simulink model "ACC_speed_change_curve_cs"  (R2016a)
settings: Solver=ode5  SolverMode=SingleTasking  StartTime=0.0  StopTime=inf  FixedStep=1/1000  RelTol=1e-3
PreLoadFcn:
  | mbxruntime.callbacks.PreLoadFcn(bdroot);
  | check_NUTS_defined;
  | 
  | assignin('base',['model_closed_' bdroot],false);addpath('../includes_ACC');
PostLoadFcn:
  | mbxruntime.callbacks.PostLoadFcn(bdroot);
InitFcn:
  | mbxruntime.callbacks.InitFcn(bdroot);
StartFcn:
  | mbxruntime.callbacks.StartFcn(bdroot);
StopFcn:
  | mbxruntime.callbacks.StopFcn(bdroot);
model workspace (MAT data in the model file):
  mbox_table : struct (value not decoded)
  model_closed = 0
  sim_status = 0
undefined symbols (not defined in the file or in its folder): DiscIntNeverNeededParam
undefined symbols (not defined in the file): SteeringColumn, SteeringWheel, WheelL0, WheelL1, WheelR0, WheelR1
libraries: simulink_extras x49, simulink x29, PreScanSimulinkLibrary x24, PreScanUsefulBlocks x2, Solver_SF x1, simulink_need_slupdate x1
(part 6 of 17)

== system ACC_speed_change_curve_cs/WheelR0_Audi_A8_1 ==
  WheelR0_Audi_A8_1 : Inport  Tag=inport/JointActuator  OutDataTypeStr=Bus: PRESCAN_POSE_DATA  SampleTime=20/1000  BusOutputAsStruct=on
  Actuator : Subsystem  Tag=VisuJoint  mask(PreScan Sink Block: VisuJoint){UniqueID=13, Translate_ObjectID3D=Audi_A8_1.WheelR0, Rotate_ObjectID3D=Audi_A8_1.WheelR0, TimeStep=20/1000, DisplayName=[]}
      mask prompts: UniqueID "Parent Unique ID"; Translate_ObjectID3D "Translate Object Name"; Rotate_ObjectID3D "Rotate Object Name"; TimeStep "Simulation Step"; DisplayName "Display Name"
      mask help:
      | The VisuJoint block provides a way to adapt the location and orientation of a part of an object.
      |
      | For more information, please click Help.
      settings: DeleteFcn=PreScanBlockDeleteFcn;
      mask Help: eval('openHelp(223)')
      mask Display: image(imread('Joint.png'))
  wires:
  WheelR0_Audi_A8_1/1 -> Actuator/1(Joint)

== system ACC_speed_change_curve_cs/WheelR0_BMW_X5_1 ==
  WheelR0_BMW_X5_1 : Inport  Tag=inport/JointActuator  OutDataTypeStr=Bus: PRESCAN_POSE_DATA  SampleTime=20/1000  BusOutputAsStruct=on
  Actuator : Subsystem  Tag=VisuJoint  mask(PreScan Sink Block: VisuJoint){UniqueID=18, Translate_ObjectID3D=BMW_X5_1.WheelR0, Rotate_ObjectID3D=BMW_X5_1.WheelR0, TimeStep=20/1000, DisplayName=[]}
      mask prompts: UniqueID "Parent Unique ID"; Translate_ObjectID3D "Translate Object Name"; Rotate_ObjectID3D "Rotate Object Name"; TimeStep "Simulation Step"; DisplayName "Display Name"
      mask help:
      | The VisuJoint block provides a way to adapt the location and orientation of a part of an object.
      |
      | For more information, please click Help.
      settings: DeleteFcn=PreScanBlockDeleteFcn;
      mask Help: eval('openHelp(223)')
      mask Display: image(imread('Joint.png'))
  wires:
  WheelR0_BMW_X5_1/1 -> Actuator/1(Joint)

== system ACC_speed_change_curve_cs/WheelR0_Toyota_Previa_1 ==
  WheelR0_Toyota_Previa_1 : Inport  Tag=inport/JointActuator  OutDataTypeStr=Bus: PRESCAN_POSE_DATA  SampleTime=20/1000  BusOutputAsStruct=on
  Actuator : Subsystem  Tag=VisuJoint  mask(PreScan Sink Block: VisuJoint){UniqueID=724, Translate_ObjectID3D=Toyota_Previa_1.WheelR0, Rotate_ObjectID3D=Toyota_Previa_1.WheelR0, TimeStep=20/1000, DisplayName=[]}
      mask prompts: UniqueID "Parent Unique ID"; Translate_ObjectID3D "Translate Object Name"; Rotate_ObjectID3D "Rotate Object Name"; TimeStep "Simulation Step"; DisplayName "Display Name"
      mask help:
      | The VisuJoint block provides a way to adapt the location and orientation of a part of an object.
      |
      | For more information, please click Help.
      settings: DeleteFcn=PreScanBlockDeleteFcn;
      mask Help: eval('openHelp(223)')
      mask Display: image(imread('Joint.png'))
  wires:
  WheelR0_Toyota_Previa_1/1 -> Actuator/1(Joint)

== system ACC_speed_change_curve_cs/WheelR0_Toyota_Yaris_1 ==
  WheelR0_Toyota_Yaris_1 : Inport  Tag=inport/JointActuator  OutDataTypeStr=Bus: PRESCAN_POSE_DATA  SampleTime=20/1000  BusOutputAsStruct=on
  Actuator : Subsystem  Tag=VisuJoint  mask(PreScan Sink Block: VisuJoint){UniqueID=721, Translate_ObjectID3D=Toyota_Yaris_1.WheelR0, Rotate_ObjectID3D=Toyota_Yaris_1.WheelR0, TimeStep=20/1000, DisplayName=[]}
      mask prompts: UniqueID "Parent Unique ID"; Translate_ObjectID3D "Translate Object Name"; Rotate_ObjectID3D "Rotate Object Name"; TimeStep "Simulation Step"; DisplayName "Display Name"
      mask help:
      | The VisuJoint block provides a way to adapt the location and orientation of a part of an object.
      |
      | For more information, please click Help.
      settings: DeleteFcn=PreScanBlockDeleteFcn;
      mask Help: eval('openHelp(223)')
      mask Display: image(imread('Joint.png'))
  wires:
  WheelR0_Toyota_Yaris_1/1 -> Actuator/1(Joint)

== system ACC_speed_change_curve_cs/WheelR1_Audi_A8_1 ==
  WheelR1_Audi_A8_1 : Inport  Tag=inport/JointActuator  OutDataTypeStr=Bus: PRESCAN_POSE_DATA  SampleTime=20/1000  BusOutputAsStruct=on
  Actuator : Subsystem  Tag=VisuJoint  mask(PreScan Sink Block: VisuJoint){UniqueID=13, Translate_ObjectID3D=Audi_A8_1.WheelR1, Rotate_ObjectID3D=Audi_A8_1.WheelR1, TimeStep=20/1000, DisplayName=[]}
      mask prompts: UniqueID "Parent Unique ID"; Translate_ObjectID3D "Translate Object Name"; Rotate_ObjectID3D "Rotate Object Name"; TimeStep "Simulation Step"; DisplayName "Display Name"
      mask help:
      | The VisuJoint block provides a way to adapt the location and orientation of a part of an object.
      |
      | For more information, please click Help.
      settings: DeleteFcn=PreScanBlockDeleteFcn;
      mask Help: eval('openHelp(223)')
      mask Display: image(imread('Joint.png'))
  wires:
  WheelR1_Audi_A8_1/1 -> Actuator/1(Joint)

== system ACC_speed_change_curve_cs/WheelR1_BMW_X5_1 ==
  WheelR1_BMW_X5_1 : Inport  Tag=inport/JointActuator  OutDataTypeStr=Bus: PRESCAN_POSE_DATA  SampleTime=20/1000  BusOutputAsStruct=on
  Actuator : Subsystem  Tag=VisuJoint  mask(PreScan Sink Block: VisuJoint){UniqueID=18, Translate_ObjectID3D=BMW_X5_1.WheelR1, Rotate_ObjectID3D=BMW_X5_1.WheelR1, TimeStep=20/1000, DisplayName=[]}
      mask prompts: UniqueID "Parent Unique ID"; Translate_ObjectID3D "Translate Object Name"; Rotate_ObjectID3D "Rotate Object Name"; TimeStep "Simulation Step"; DisplayName "Display Name"
      mask help:
      | The VisuJoint block provides a way to adapt the location and orientation of a part of an object.
      |
      | For more information, please click Help.
      settings: DeleteFcn=PreScanBlockDeleteFcn;
      mask Help: eval('openHelp(223)')
      mask Display: image(imread('Joint.png'))
  wires:
  WheelR1_BMW_X5_1/1 -> Actuator/1(Joint)

== system ACC_speed_change_curve_cs/WheelR1_Toyota_Previa_1 ==
  WheelR1_Toyota_Previa_1 : Inport  Tag=inport/JointActuator  OutDataTypeStr=Bus: PRESCAN_POSE_DATA  SampleTime=20/1000  BusOutputAsStruct=on
  Actuator : Subsystem  Tag=VisuJoint  mask(PreScan Sink Block: VisuJoint){UniqueID=724, Translate_ObjectID3D=Toyota_Previa_1.WheelR1, Rotate_ObjectID3D=Toyota_Previa_1.WheelR1, TimeStep=20/1000, DisplayName=[]}
      mask prompts: UniqueID "Parent Unique ID"; Translate_ObjectID3D "Translate Object Name"; Rotate_ObjectID3D "Rotate Object Name"; TimeStep "Simulation Step"; DisplayName "Display Name"
      mask help:
      | The VisuJoint block provides a way to adapt the location and orientation of a part of an object.
      |
      | For more information, please click Help.
      settings: DeleteFcn=PreScanBlockDeleteFcn;
      mask Help: eval('openHelp(223)')
      mask Display: image(imread('Joint.png'))
  wires:
  WheelR1_Toyota_Previa_1/1 -> Actuator/1(Joint)

== system ACC_speed_change_curve_cs/WheelR1_Toyota_Yaris_1 ==
  WheelR1_Toyota_Yaris_1 : Inport  Tag=inport/JointActuator  OutDataTypeStr=Bus: PRESCAN_POSE_DATA  SampleTime=20/1000  BusOutputAsStruct=on
  Actuator : Subsystem  Tag=VisuJoint  mask(PreScan Sink Block: VisuJoint){UniqueID=721, Translate_ObjectID3D=Toyota_Yaris_1.WheelR1, Rotate_ObjectID3D=Toyota_Yaris_1.WheelR1, TimeStep=20/1000, DisplayName=[]}
      mask prompts: UniqueID "Parent Unique ID"; Translate_ObjectID3D "Translate Object Name"; Rotate_ObjectID3D "Rotate Object Name"; TimeStep "Simulation Step"; DisplayName "Display Name"
      mask help:
      | The VisuJoint block provides a way to adapt the location and orientation of a part of an object.
      |
      | For more information, please click Help.
      settings: DeleteFcn=PreScanBlockDeleteFcn;
      mask Help: eval('openHelp(223)')
      mask Display: image(imread('Joint.png'))
  wires:
  WheelR1_Toyota_Yaris_1/1 -> Actuator/1(Joint)

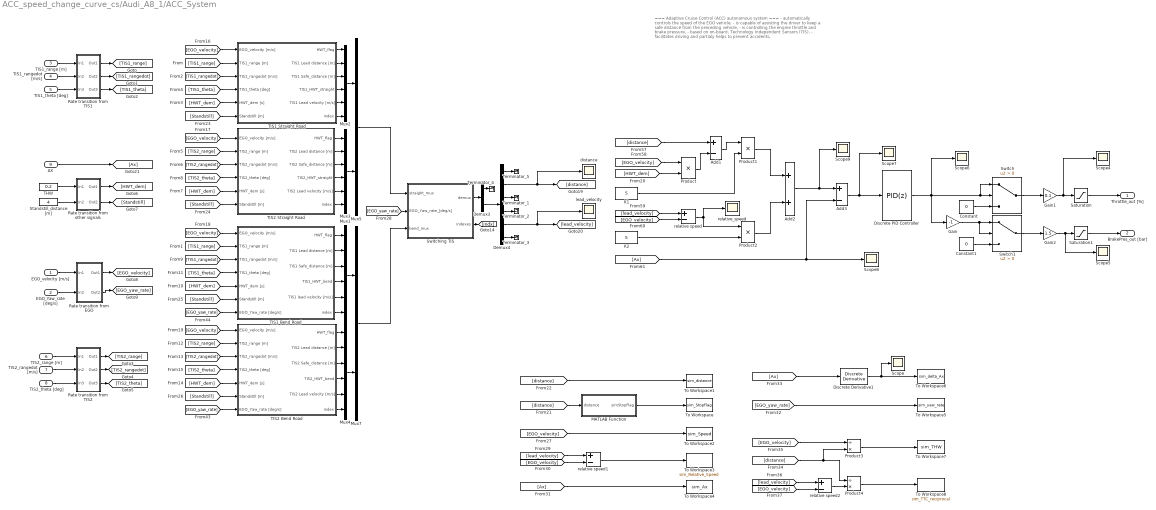
== system ACC_speed_change_curve_cs/Audi_A8_1/ACC_System ==
  note: === Adaptive Cruise Control (ACC) autonomous system ===
      |
      |  - automatically controls the speed of the EGO vehicle,
      |  - is capable of assisting the driver to keep a safe distance
      |    from the preceding vehicle,
      |  - is controlling the engine throttle and brake pressure,
      |  - based on on-board, Technology Independent Sensors (TIS),
      |  - facilitates driving and partialy helps to prevent accidents.
  EGO_velocity [m/s] : Inport  SampleTime=Tblock
  EGO_Yaw_rate [deg/s] : Inport  Port=2  SampleTime=Tblock
  TIS1_range [m] : Inport  Port=3  PortDimensions=TISdet(1)  SampleTime=TISsensor(1)
  TIS1_rangedot [m/s] : Inport  Port=4  PortDimensions=TISdet(1)  SampleTime=TISsensor(1)
  TIS1_theta [deg] : Inport  Port=5  PortDimensions=TISdet(1)  SampleTime=TISsensor(1)
  TIS2_range [m] : Inport  Port=6  PortDimensions=TISdet(2)  SampleTime=TISsensor(2)
  TIS2_rangedot [m/s] : Inport  Port=7  PortDimensions=TISdet(2)  SampleTime=TISsensor(2)
  TIS2_theta [deg] : Inport  Port=8  PortDimensions=TISdet(2)  SampleTime=TISsensor(2)
  AX : Inport  Port=9
  Add1 : Sum  Inputs=+-
  Add2 : Sum
  Add3 : Sum  Inputs=+-
  Constant : Constant  Value=0
  Constant1 : Constant  Value=0
  Demux3 : Demux  Outputs=2
  Demux4 : Demux  Outputs=6
  Discrete Derivative1 : simulink/Discrete/Discrete Derivative  gainval=1.0  ICPrevScaledInput=0.0  OutMin=[]  OutMax=[]  OutDataType=fixdt(1, 16)  OutScaling=2^-10  DoSatur=off
  Discrete PID Controller : simulink/Continuous/PID Controller  Controller=PID  TimeDomain=Discrete-time  SampleTime=-1  IntegratorMethod=Forward Euler  FilterMethod=Forward Euler  Form=Parallel  UseFilter=on  ControllerParametersSource=internal  P=50  I=5  D=0  N=100  InitialConditionSource=internal  InitialConditionForIntegrator=0  InitialConditionForFilter=0  ExternalReset=none  LimitOutput=off  UpperSaturationLimit=inf  LowerSaturationLimit=-inf  LinearizeAsGain=off  AntiWindupMode=none  Kb=1  TrackingMode=off  Kt=1  PParamMin=[]  PParamMax=[]  IParamMin=[]  IParamMax=[]  DParamMin=[]  DParamMax=[]  NParamMin=[]  NParamMax=[]  KbParamMin=[]  KbParamMax=[]  KtParamMin=[]  KtParamMax=[]  POutMin=[]  POutMax=[]  IOutMin=[]  IOutMax=[]  DOutMin=[]  DOutMax=[]  NOutMin=[]  NOutMax=[]  KbOutMin=[]  KbOutMax=[]  KtOutMin=[]  KtOutMax=[]  IntegratorOutMin=[]  IntegratorOutMax=[]  FilterOutMin=[]  FilterOutMax=[]  SumOutMin=[]  SumOutMax=[]  SumI1OutMin=[]  SumI1OutMax=[]  SumI2OutMin=[]  SumI2OutMax=[]  SumI3OutMin=[]  SumI3OutMax=[]  SumDOutMin=[]  SumDOutMax=[]  SaturationOutMin=[]  SaturationOutMax=[]  IntegratorContinuousStateAttributes=''  IntegratorStateMustResolveToSignalObject=off  IntegratorRTWStateStorageClass=Auto  FilterContinuousStateAttributes=''  FilterStateMustResolveToSignalObject=off  FilterRTWStateStorageClass=Auto  DifferentiatorICPrevScaledInput=0  DifferentiatorOutMin=[]  DifferentiatorOutMax=[]
  Gain : Gain  Gain=-1
  Gain1 : Gain  Gain=0.1
  Gain2 : Gain  Gain=1.5
  K1 : Constant  Value=5
  K2 : Constant  Value=5
  MATLAB Function : MATLAB Function  TreatAsAtomicUnit=on
  Mux{1..4} (4 alike) : Mux  Inputs=6
  Mux5 : Mux  Inputs=2
  Mux7 : Mux  Inputs=2
  Product : Product
  Product1 : Product
  Product2 : Product
  Product3 : Product  Inputs=/*
  Product4 : Product  Inputs=/*
  Rate transition from other signals : Subsystem
  Rate transition from EGO : Subsystem
  Rate transition from TIS1 : Subsystem
  Rate transition from TIS2 : Subsystem
  Saturation : Saturate  UpperLimit=100  LowerLimit=0
  Saturation1 : Saturate  UpperLimit=120  LowerLimit=0
  Scope{,4..9} (7 alike) : Scope
  Standstill_distance [m] : Constant  Value=4
  Switch : Switch  Criteria=u2 > Threshold
  Switch1 : Switch  Criteria=u2 > Threshold
  Switching TIS : Subsystem
  THW : Constant  Value=0.2
  TIS1 Bend Road : Subsystem
  TIS1 Straight Road : Subsystem
  TIS2 Bend Road : Subsystem
  TIS2 Straight Road : Subsystem
  Terminator_{1..5} (5 alike) : Terminator
  To Workspace : ToWorkspace  VariableName=sim_StopFlag  SampleTime=-1
  To Workspace1 : ToWorkspace  VariableName=sim_distance  SaveFormat=Structure With Time  SampleTime=-1
  To Workspace2 : ToWorkspace  VariableName=sim_Speed  SaveFormat=Structure With Time  SampleTime=-1
  To Workspace3 : ToWorkspace  VariableName=sim_Relative_Speed  SaveFormat=Structure With Time  SampleTime=-1
  To Workspace4 : ToWorkspace  VariableName=sim_Ax  SaveFormat=Structure With Time  SampleTime=-1
  To Workspace5 : ToWorkspace  VariableName=sim_yaw_rate  SaveFormat=Structure With Time  SampleTime=-1
  To Workspace6 : ToWorkspace  VariableName=sim_delta_Ax  SaveFormat=Structure With Time  SampleTime=-1
  To Workspace7 : ToWorkspace  VariableName=sim_THW  SaveFormat=Structure With Time  SampleTime=-1
  To Workspace8 : ToWorkspace  VariableName=sim_TTC_reciprocal  SaveFormat=Structure With Time  SampleTime=-1
  distance : Scope
  lead_velocity : Scope
  relative speed : Sum  Inputs=+-
  relative speed1 : Sum  Inputs=+-
  relative speed2 : Sum  Inputs=+-
  relative_speed : Scope
  Throttle_out [%] : Outport
  BrakePres_out [bar] : Outport  Port=2
  wires:
  TIS1 Straight Road/1(HWT_flag) -> Mux2/1
  TIS1 Straight Road/2(TIS1 Lead distance [m]) -> Mux2/2
  TIS1 Straight Road/3(TIS1 Safe_distance [m]) -> Mux2/3
  TIS1 Straight Road/4(TIS1_HWT_straight) -> Mux2/4
  TIS1 Straight Road/5(TIS1 Lead velocity [m/s]) -> Mux2/5
  TIS1 Straight Road/6(index) -> Mux2/6
  TIS1_range [m]/1 -> Rate transition from TIS1/1(In1)
  TIS1_rangedot [m/s]/1 -> Rate transition from TIS1/2(In2)
  TIS1_theta [deg]/1 -> Rate transition from TIS1/3(In3)
  TIS2_range [m]/1 -> Rate transition from TIS2/1(In1)
  TIS2_rangedot [m/s]/1 -> Rate transition from TIS2/2(In2)
  TIS2_theta [deg]/1 -> Rate transition from TIS2/3(In3)
  Rate transition from TIS1/1(Out1) -> [TIS1_range]
  Rate transition from TIS1/2(Out2) -> [TIS1_rangedot]
  Rate transition from TIS1/3(Out3) -> [TIS1_theta]
  Rate transition from TIS2/1(Out1) -> [TIS2_range]
  Rate transition from TIS2/2(Out2) -> [TIS2_rangedot]
  Rate transition from TIS2/3(Out3) -> [TIS2_theta]
  [TIS1_range] -> TIS1 Straight Road/2(TIS1_range [m])
  [TIS1_rangedot] -> TIS1 Straight Road/3(TIS1_rangedot [m/s])
  [TIS1_theta] -> TIS1 Straight Road/4(TIS1_theta [deg])
  [TIS2_range] -> TIS2 Straight Road/2(TIS2_range [m])
  [TIS2_rangedot] -> TIS2 Straight Road/3(TIS2_rangedot [m/s])
  [TIS2_theta] -> TIS2 Straight Road/4(TIS2_theta [deg])
  [TIS1_range] -> TIS1 Bend Road/2(TIS1_range [m])
  [TIS1_rangedot] -> TIS1 Bend Road/3(TIS1_rangedot [m/s])
  [TIS1_theta] -> TIS1 Bend Road/4(TIS1_theta [deg])
  [TIS2_range] -> TIS2 Bend Road/2(TIS2_range [m])
  [TIS2_rangedot] -> TIS2 Bend Road/3(TIS2_rangedot [m/s])
  [TIS2_theta] -> TIS2 Bend Road/4(TIS2_theta [deg])
  EGO_velocity [m/s]/1 -> Rate transition from EGO/1(In1)
  EGO_Yaw_rate [deg/s]/1 -> Rate transition from EGO/2(In2)
  THW/1 -> Rate transition from other signals/1(In1)
  Standstill_distance [m]/1 -> Rate transition from other signals/2(In2)
  Rate transition from other signals/1(Out1) -> [HWT_dem]
  Rate transition from other signals/2(Out2) -> [Standstill]
  [HWT_dem] -> TIS1 Straight Road/5(HWT_dem [s])
  [HWT_dem] -> TIS2 Straight Road/5(HWT_dem [s])
  [HWT_dem] -> TIS1 Bend Road/5(HWT_dem [s])
  [HWT_dem] -> TIS2 Bend Road/5(HWT_dem [s])
  Rate transition from EGO/1(Out1) -> [EGO_velocity]
  Rate transition from EGO/2(Out2) -> [EGO_yaw_rate]
  [EGO_velocity] -> TIS1 Straight Road/1(EGO_velocity [m/s])
  [EGO_velocity] -> TIS2 Straight Road/1(EGO_velocity [m/s])
  [EGO_velocity] -> TIS1 Bend Road/1(EGO_velocity [m/s])
  [EGO_velocity] -> TIS2 Bend Road/1(EGO_velocity [m/s])
  [Standstill] -> TIS1 Straight Road/6(Standstill [m])
  [Standstill] -> TIS2 Straight Road/6(Standstill [m])
  [Standstill] -> TIS1 Bend Road/6(Standstill [m])
  [Standstill] -> TIS2 Bend Road/6(Standstill [m])
  [EGO_yaw_rate] -> Switching TIS/2(EGO_Yaw_rate_[deg/s])
  [EGO_yaw_rate] -> TIS2 Bend Road/7(EGO_Yaw_rate [deg/s])
  [EGO_yaw_rate] -> TIS1 Bend Road/7(EGO_Yaw_rate [deg/s])
  Mux2/1 -> Mux5/1
  TIS2 Straight Road/1(HWT_flag) -> Mux3/1
  TIS2 Straight Road/2(TIS2 Lead distance [m]) -> Mux3/2
  TIS2 Straight Road/3(TIS2 Safe_distance [m]) -> Mux3/3
  TIS2 Straight Road/4(TIS2_HWT_straight) -> Mux3/4
  TIS2 Straight Road/5(TIS2 Lead velocity [m/s]) -> Mux3/5
  TIS2 Straight Road/6(index) -> Mux3/6
  Mux3/1 -> Mux5/2
  TIS2 Bend Road/1(HWT_flag) -> Mux4/1
  TIS2 Bend Road/2(TIS2 Lead distance [m]) -> Mux4/2
  TIS2 Bend Road/3(TIS2 Safe_distance [m]) -> Mux4/3
  TIS2 Bend Road/4(TIS2_HWT_bend) -> Mux4/4
  TIS2 Bend Road/5(TIS2 Lead velocity [m/s]) -> Mux4/5
  TIS2 Bend Road/6(index) -> Mux4/6
  Mux5/1 -> Switching TIS/1(straight_mux)
  TIS1 Bend Road/1(HWT_flag) -> Mux1/1
  TIS1 Bend Road/2(TIS1 Lead distance [m]) -> Mux1/2
  TIS1 Bend Road/3(TIS1 Safe_distance [m]) -> Mux1/3
  TIS1 Bend Road/4(TIS1_HWT_bend) -> Mux1/4
  TIS1 Bend Road/5(TIS1 lead velocity [m/s]) -> Mux1/5
  TIS1 Bend Road/6(index) -> Mux1/6
  Mux1/1 -> Mux7/1
  Mux4/1 -> Mux7/2
  Mux7/1 -> Switching TIS/3(bend_mux)
  Switching TIS/2(indexes) -> [indx]
  Switching TIS/1(demux) -> Demux3/1
  Demux4/2 -> [distance], distance/1
  Demux4/5 -> lead_velocity/1, [lead_velocity]
  Demux3/2 -> Demux4/1
  [lead_velocity] -> relative speed/1
  [EGO_velocity] -> relative speed/2
  AX/1 -> [Ax]
  [EGO_velocity] -> Product/1
  [HWT_dem] -> Product/2
  Product/1 -> Add1/2
  [distance] -> Add1/1
  K1/1 -> Product1/2
  Add1/1 -> Product1/1
  Product1/1 -> Add2/1
  relative speed/1 -> Product2/1, relative_speed/1
  K2/1 -> Product2/2
  Product2/1 -> Add2/2
  Add2/1 -> Scope9/1, Add3/1
  Add3/1 -> Scope7/1, Discrete PID Controller/1
  Constant/1 -> Switch/3
  Constant1/1 -> Switch1/3
  Gain/1 -> Switch1/1, Switch1/2
  Switch/1 -> Gain1/1
  Gain1/1 -> Scope4/1, Saturation/1
  Switch1/1 -> Gain2/1
  Gain2/1 -> Scope5/1, Saturation1/1
  Saturation/1 -> Throttle_out [%]/1
  Saturation1/1 -> BrakePres_out [bar]/1
  Discrete PID Controller/1 -> Gain/1, Switch/1, Switch/2, Scope6/1
  Demux4/1 -> Terminator_5/1
  Demux4/3 -> Terminator_1/1
  Demux4/4 -> Terminator_2/1
  Demux4/6 -> Terminator_3/1
  Demux3/1 -> Terminator_4/1
  MATLAB Function/1(simStopFlag) -> To Workspace/1
  [distance] -> MATLAB Function/1(distance)
  [Ax] -> Scope8/1, Add3/2
  [distance] -> To Workspace1/1
  [EGO_velocity] -> To Workspace2/1
  [lead_velocity] -> relative speed1/1
  [EGO_velocity] -> relative speed1/2
  relative speed1/1 -> To Workspace3/1
  [Ax] -> To Workspace4/1
  [Ax] -> Discrete Derivative1/1
  [EGO_yaw_rate] -> To Workspace5/1
  [lead_velocity] -> relative speed2/1
  [EGO_velocity] -> relative speed2/2
  [EGO_velocity] -> Product3/1
  [distance] -> Product4/1, Product3/2
  relative speed2/1 -> Product4/2
  Product3/1 -> To Workspace7/1
  Product4/1 -> To Workspace8/1
  Discrete Derivative1/1 -> To Workspace6/1, Scope/1

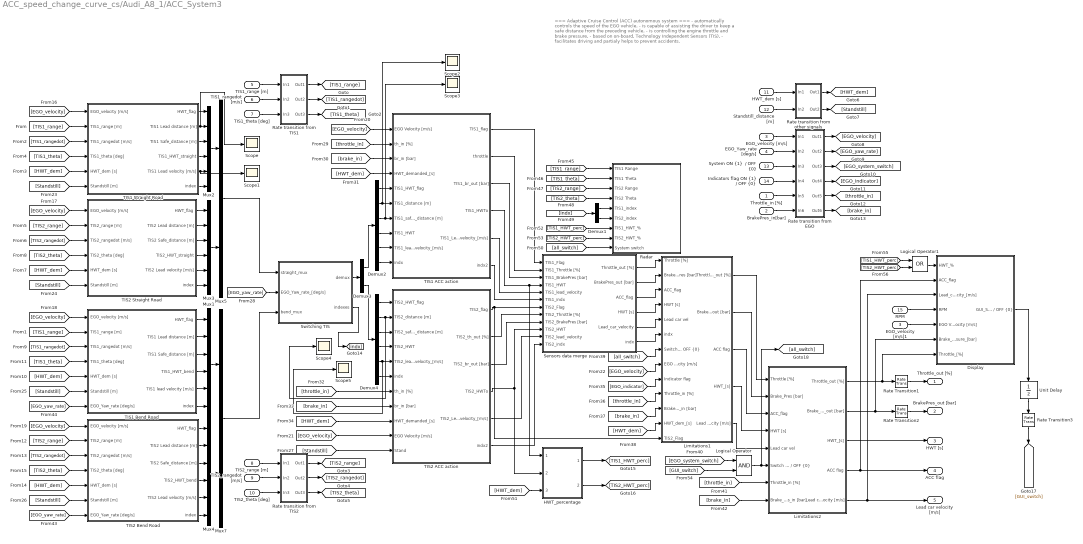
== system ACC_speed_change_curve_cs/Audi_A8_1/ACC_System3 ==
  note: === Adaptive Cruise Control (ACC) autonomous system ===
      |
      |  - automatically controls the speed of the EGO vehicle,
      |  - is capable of assisting the driver to keep a safe distance
      |    from the preceding vehicle,
      |  - is controlling the engine throttle and brake pressure,
      |  - based on on-board, Technology Independent Sensors (TIS),
      |  - facilitates driving and partialy helps to prevent accidents.
  Throttle_in [%] : Inport  SampleTime=0
  BrakePres_in[bar] : Inport  Port=2  SampleTime=0
  EGO_velocity [m/s] : Inport  Port=3  SampleTime=Tblock
  EGO_Yaw_rate [deg/s] : Inport  Port=4  SampleTime=Tblock
  TIS1_range [m] : Inport  Port=5  PortDimensions=TISdet(1)  SampleTime=TISsensor(1)
  TIS1_rangedot [m/s] : Inport  Port=6  PortDimensions=TISdet(1)  SampleTime=TISsensor(1)
  TIS1_theta [deg] : Inport  Port=7  PortDimensions=TISdet(1)  SampleTime=TISsensor(1)
  TIS2_range [m] : Inport  Port=8  PortDimensions=TISdet(2)  SampleTime=TISsensor(2)
  TIS2_rangedot [m/s] : Inport  Port=9  PortDimensions=TISdet(2)  SampleTime=TISsensor(2)
  TIS2_theta [deg] : Inport  Port=10  PortDimensions=TISdet(2)  SampleTime=TISsensor(2)
  HWT_dem [s] : Inport  Port=11
  Standstill_distance [m] : Inport  Port=12
  "System ON {1}  / OFF {0}" : Inport  Port=13
  "Indicators flag ON {1} / OFF {0}" : Inport  Port=14
  RPM : Inport  Port=15  SampleTime=0
  Demux1 : Demux  Outputs=2
  Demux2 : Demux  Outputs=6
  Demux3 : Demux  Outputs=2
  Demux4 : Demux  Outputs=6
  Display : Subsystem
  EGO_velocity [m/s]1 : InportShadow  Port=3  SampleTime=Tblock
  HWT_percentage : Subsystem
  Limitations1 : Subsystem
  Limitations2 : Subsystem
  Logical Operator : Logic  AllPortsSameDT=off  OutDataTypeStr=boolean
  Logical Operator1 : Logic  Operator=OR  AllPortsSameDT=off  OutDataTypeStr=boolean
  Mux{1..4} (4 alike) : Mux  Inputs=6
  Mux5 : Mux  Inputs=2
  Mux7 : Mux  Inputs=2
  Radar : Subsystem
  Rate Transition1 : RateTransition  Integrity=off  OutPortSampleTime=0
  Rate Transition2 : RateTransition  Integrity=off  OutPortSampleTime=0
  Rate Transition3 : RateTransition  Integrity=off  OutPortSampleTime=Tsensor
  Rate transition from other signals : Subsystem
  Rate transition from EGO : Subsystem
  Rate transition from TIS1 : Subsystem
  Rate transition from TIS2 : Subsystem
  Scope{,1..5} (6 alike) : Scope
  Sensors data merge : Subsystem
  Switching TIS : Subsystem
  TIS1 ACC action : Subsystem
  TIS1 Bend Road : Subsystem
  TIS1 Straight Road : Subsystem
  TIS2 ACC action : Subsystem
  TIS2 Bend Road : Subsystem
  TIS2 Straight Road : Subsystem
  Unit Delay : UnitDelay  InitialCondition=1  SampleTime=-1
  Throttle_out [%] : Outport
  BrakePres_out [bar] : Outport  Port=2
  HWT [s] : Outport  Port=3
  ACC flag : Outport  Port=4
  Lead car velocity [m/s] : Outport  Port=5
  wires:
  Logical Operator1/1 -> Display/1(HWT_%)
  [TIS2_HWT_perc] -> Logical Operator1/2
  [TIS1_HWT_perc] -> Logical Operator1/1
  [all_switch] -> Radar/9(System switch)
  [GUI_switch] -> Logical Operator/2
  [EGO_system_switch] -> Logical Operator/1
  Logical Operator/1 -> [all_switch], Limitations2/6("Switch ON {1} / OFF {0}")
  Rate Transition3/1 -> [GUI_switch]
  Unit Delay/1 -> Rate Transition3/1
  EGO_velocity [m/s]1/1 -> Display/5(EGO Velocity [m/s])
  RPM/1 -> Display/4(RPM)
  Display/1("GUI_System ON {1} / OFF {0}") -> Unit Delay/1
  [TIS2_HWT_perc] -> Radar/8(TIS2_HWT_%)
  [TIS1_HWT_perc] -> Radar/7(TIS1_HWT_%)
  HWT_percentage/2(TIS2_HWT_perc) -> [TIS2_HWT_perc]
  HWT_percentage/1(TIS1_HWT_perc) -> [TIS1_HWT_perc]
  [HWT_dem] -> HWT_percentage/3(HWT_dem_[s])
  Demux3/2 -> Demux4/1
  Demux4/6 -> TIS2 ACC action/6(indx)
  Demux4/5 -> Scope5/1, TIS2 ACC action/5(TIS2_lead_velocity_[m/s])
  Demux4/4 -> TIS2 ACC action/4(TIS2_HWT)
  Demux4/3 -> TIS2 ACC action/3(TIS2_safe_distance [m])
  Demux4/2 -> Scope4/1, TIS2 ACC action/2(TIS2_distance [m])
  Demux4/1 -> TIS2 ACC action/1(TIS2_HWT_flag)
  Demux3/1 -> Demux2/1
  Demux2/6 -> TIS1 ACC action/10(indx)
  Demux2/5 -> TIS1 ACC action/9(TIS1_lead_velocity_[m/s])
  Demux2/4 -> TIS1 ACC action/8(TIS1_HWT)
  Demux2/3 -> Scope3/1, TIS1 ACC action/7(TIS1_safe_distance [m])
  Demux2/2 -> Scope2/1, TIS1 ACC action/6(TIS1_distance [m])
  Demux2/1 -> TIS1 ACC action/5(TIS1_HWT_flag)
  Switching TIS/1(demux) -> Demux3/1
  [indx] -> Demux1/1
  Demux1/2 -> Radar/6(TIS2_index)
  Demux1/1 -> Radar/5(TIS1_index)
  Switching TIS/2(indexes) -> [indx]
  Mux7/1 -> Switching TIS/3(bend_mux)
  Mux4/1 -> Mux7/2
  Mux1/1 -> Mux7/1
  TIS1 Bend Road/6(index) -> Mux1/6
  TIS1 Bend Road/5(TIS1 lead velocity [m/s]) -> Mux1/5
  TIS1 Bend Road/4(TIS1_HWT_bend) -> Mux1/4
  TIS1 Bend Road/3(TIS1 Safe_distance [m]) -> Mux1/3
  TIS1 Bend Road/2(TIS1 Lead distance [m]) -> Mux1/2
  TIS1 Bend Road/1(HWT_flag) -> Mux1/1
  Mux5/1 -> Switching TIS/1(straight_mux)
  TIS2 Bend Road/6(index) -> Mux4/6
  TIS2 Bend Road/5(TIS2 Lead velocity [m/s]) -> Mux4/5
  TIS2 Bend Road/4(TIS2_HWT_bend) -> Mux4/4
  TIS2 Bend Road/3(TIS2 Safe_distance [m]) -> Mux4/3
  TIS2 Bend Road/2(TIS2 Lead distance [m]) -> Mux4/2
  TIS2 Bend Road/1(HWT_flag) -> Mux4/1
  Mux3/1 -> Mux5/2
  TIS2 Straight Road/6(index) -> Mux3/6
  TIS2 Straight Road/5(TIS2 Lead velocity [m/s]) -> Mux3/5
  TIS2 Straight Road/4(TIS2_HWT_straight) -> Mux3/4
  TIS2 Straight Road/3(TIS2 Safe_distance [m]) -> Mux3/3
  TIS2 Straight Road/2(TIS2 Lead distance [m]) -> Mux3/2
  TIS2 Straight Road/1(HWT_flag) -> Mux3/1
  Mux2/1 -> Mux5/1
  [TIS2_theta] -> Radar/4(TIS2 Theta)
  [TIS2_range] -> Radar/3(TIS2 Range)
  [TIS1_theta] -> Radar/2(TIS1 Theta)
  [TIS1_range] -> Radar/1(TIS1 Range)
  Limitations2/5(Lead car velocity [m/s]) -> Display/3(Lead_car_velocity_[m/s]), Lead car velocity [m/s]/1
  Limitations2/4(ACC flag) -> Display/2(ACC_flag), ACC flag/1
  Limitations2/3(HWT_[s]) -> HWT [s]/1
  Rate Transition2/1 -> BrakePres_out [bar]/1
  Rate Transition1/1 -> Throttle_out [%]/1
  Limitations2/2(Brake_Pres_out [bar]) -> Display/6(Brake_Pressure_[bar]), Rate Transition2/1
  Limitations2/1(Throttle_out [%]) -> Display/7(Throttle_[%]), Rate Transition1/1
  [EGO_yaw_rate] -> TIS1 Bend Road/7(EGO_Yaw_rate [deg/s])
  [EGO_yaw_rate] -> TIS2 Bend Road/7(EGO_Yaw_rate [deg/s])
  [brake_in] -> Limitations2/8(Brake_Pres_in [bar])
  [throttle_in] -> Limitations2/7(Throttle_in [%])
  [all_switch] -> Limitations1/7("Switch ON {1} / OFF {0}")
  [HWT_dem] -> Limitations1/12(HWT_dem_[s])
  [brake_in] -> Limitations1/11(Brake_Pres_in [bar])
  [throttle_in] -> Limitations1/10(Throttle_in [%])
  [EGO_indicator] -> Limitations1/9(Indicator flag)
  [HWT_dem] -> TIS2 ACC action/9(HWT_demanded_[s])
  [brake_in] -> TIS2 ACC action/8(br_in [bar])
  [throttle_in] -> TIS2 ACC action/7(th_in [%])
  [HWT_dem] -> TIS1 ACC action/4(HWT_demanded_[s])
  [brake_in] -> TIS1 ACC action/3(br_in [bar])
  [throttle_in] -> TIS1 ACC action/2(th_in [%])
  [EGO_yaw_rate] -> Switching TIS/2(EGO_Yaw_rate_[deg/s])
  [Standstill] -> TIS2 ACC action/11(Stand)
  [Standstill] -> TIS2 Bend Road/6(Standstill [m])
  [Standstill] -> TIS1 Bend Road/6(Standstill [m])
  [Standstill] -> TIS2 Straight Road/6(Standstill [m])
  [Standstill] -> TIS1 Straight Road/6(Standstill [m])
  [EGO_velocity] -> Limitations1/8(EGO Velocity [m/s])
  [EGO_velocity] -> TIS2 ACC action/10(EGO Velocity [m/s])
  [EGO_velocity] -> TIS1 ACC action/1(EGO Velocity [m/s])
  [EGO_velocity] -> TIS2 Bend Road/1(EGO_velocity [m/s])
  [EGO_velocity] -> TIS1 Bend Road/1(EGO_velocity [m/s])
  [EGO_velocity] -> TIS2 Straight Road/1(EGO_velocity [m/s])
  [EGO_velocity] -> TIS1 Straight Road/1(EGO_velocity [m/s])
  Rate transition from EGO/6(Out6) -> [brake_in]
  Rate transition from EGO/5(Out5) -> [throttle_in]
  Rate transition from EGO/4(Out4) -> [EGO_indicator]
  Rate transition from EGO/3(Out3) -> [EGO_system_switch]
  Rate transition from EGO/2(Out2) -> [EGO_yaw_rate]
  Rate transition from EGO/1(Out1) -> [EGO_velocity]
  [HWT_dem] -> TIS2 Bend Road/5(HWT_dem [s])
  [HWT_dem] -> TIS1 Bend Road/5(HWT_dem [s])
  [HWT_dem] -> TIS2 Straight Road/5(HWT_dem [s])
  [HWT_dem] -> TIS1 Straight Road/5(HWT_dem [s])
  Rate transition from other signals/2(Out2) -> [Standstill]
  Rate transition from other signals/1(Out1) -> [HWT_dem]
  "Indicators flag ON {1} / OFF {0}"/1 -> Rate transition from EGO/4(In4)
  BrakePres_in[bar]/1 -> Rate transition from EGO/6(In6)
  Throttle_in [%]/1 -> Rate transition from EGO/5(In5)
  "System ON {1}  / OFF {0}"/1 -> Rate transition from EGO/3(In3)
  Standstill_distance [m]/1 -> Rate transition from other signals/2(In2)
  HWT_dem [s]/1 -> Rate transition from other signals/1(In1)
  EGO_Yaw_rate [deg/s]/1 -> Rate transition from EGO/2(In2)
  EGO_velocity [m/s]/1 -> Rate transition from EGO/1(In1)
  [TIS2_theta] -> TIS2 Bend Road/4(TIS2_theta [deg])
  [TIS2_rangedot] -> TIS2 Bend Road/3(TIS2_rangedot [m/s])
  [TIS2_range] -> TIS2 Bend Road/2(TIS2_range [m])
  [TIS1_theta] -> TIS1 Bend Road/4(TIS1_theta [deg])
  [TIS1_rangedot] -> TIS1 Bend Road/3(TIS1_rangedot [m/s])
  [TIS1_range] -> TIS1 Bend Road/2(TIS1_range [m])
  [TIS2_theta] -> TIS2 Straight Road/4(TIS2_theta [deg])
  [TIS2_rangedot] -> TIS2 Straight Road/3(TIS2_rangedot [m/s])
  [TIS2_range] -> TIS2 Straight Road/2(TIS2_range [m])
  [TIS1_theta] -> TIS1 Straight Road/4(TIS1_theta [deg])
  [TIS1_rangedot] -> TIS1 Straight Road/3(TIS1_rangedot [m/s])
  [TIS1_range] -> TIS1 Straight Road/2(TIS1_range [m])
  Rate transition from TIS2/3(Out3) -> [TIS2_theta]
  Rate transition from TIS2/2(Out2) -> [TIS2_rangedot]
  Rate transition from TIS2/1(Out1) -> [TIS2_range]
  Rate transition from TIS1/3(Out3) -> [TIS1_theta]
  Rate transition from TIS1/2(Out2) -> [TIS1_rangedot]
  Rate transition from TIS1/1(Out1) -> [TIS1_range]
  TIS2_theta [deg]/1 -> Rate transition from TIS2/3(In3)
  TIS2_rangedot [m/s]/1 -> Rate transition from TIS2/2(In2)
  TIS2_range [m]/1 -> Rate transition from TIS2/1(In1)
  TIS1_theta [deg]/1 -> Rate transition from TIS1/3(In3)
  TIS1_rangedot [m/s]/1 -> Rate transition from TIS1/2(In2)
  TIS1_range [m]/1 -> Rate transition from TIS1/1(In1)
  Limitations1/5(Lead car velocity [m/s]) -> Limitations2/5(Lead car vel)
  Limitations1/3(ACC flag) -> Limitations2/3(ACC_flag)
  Limitations1/4(HWT_[s]) -> Limitations2/4(HWT [s])
  Limitations1/2(Brake_Pres_out [bar]) -> Limitations2/2(Brake_Pres [bar])
  Limitations1/1(Throttle_out [%]) -> Limitations2/1(Throttle [%])
  Sensors data merge/6(indx) -> Limitations1/6(indx)
  TIS2 ACC action/6(indx2) -> Sensors data merge/12(TIS2_indx)
  TIS1 ACC action/6(indx2) -> Sensors data merge/6(TIS1_indx)
  TIS1 Straight Road/6(index) -> Mux2/6
  TIS1 Straight Road/5(TIS1 Lead velocity [m/s]) -> Mux2/5, Scope1/1
  TIS1 Straight Road/4(TIS1_HWT_straight) -> Mux2/4
  TIS1 Straight Road/3(TIS1 Safe_distance [m]) -> Mux2/3
  TIS1 Straight Road/2(TIS1 Lead distance [m]) -> Mux2/2, Scope/1
  TIS1 Straight Road/1(HWT_flag) -> Mux2/1
  TIS2 ACC action/5(TIS2_Lead_velocity_[m/s]) -> Sensors data merge/11(TIS2_lead_velocity)
  TIS2 ACC action/4(TIS2_HWTo) -> HWT_percentage/2(TIS2_HWT), Sensors data merge/10(TIS2_HWT)
  TIS2 ACC action/3(TIS2_br_out [bar]) -> Sensors data merge/9(TIS2_BrakePres [bar])
  TIS2 ACC action/2(TIS2_th_out [%]) -> Sensors data merge/8(TIS2_Throttle [%])
  TIS2 ACC action/1(TIS2_flag) -> Limitations1/13(TIS2_Flag), Sensors data merge/7(TIS2_Flag)
  TIS1 ACC action/5(TIS1_Lead_velocity_[m/s]) -> Sensors data merge/5(TIS1_lead_velocity)
  Sensors data merge/5(Lead_car_velocity) -> Limitations1/5(Lead car vel)
  Sensors data merge/4(HWT [s]) -> Limitations1/4(HWT [s])
  Sensors data merge/3(ACC_flag) -> Limitations1/3(ACC_flag)
  TIS1 ACC action/4(TIS1_HWTo) -> HWT_percentage/1(TIS1_HWT), Sensors data merge/4(TIS1_HWT)
  TIS1 ACC action/3(TIS1_br_out [bar]) -> Sensors data merge/3(TIS1_BrakePres [bar])
  TIS1 ACC action/2(throttle) -> Sensors data merge/2(TIS1_Throttle [%])
  TIS1 ACC action/1(TIS1_flag) -> Sensors data merge/1(TIS1_Flag)
  Sensors data merge/2(BrakePres_out [bar]) -> Limitations1/2(Brake_Pres [bar])
  Sensors data merge/1(Throttle_out [%]) -> Limitations1/1(Throttle [%])

== system ACC_speed_change_curve_cs/Audi_A8_1/Brake_light_left_Mux ==
  MSCD [Cd] : Inport
  Position (xyz) [m] : Inport  Port=2
  Orientation (RPY) [deg] : Inport  Port=3
  Color [-] : Inport  Port=4
  TextureResourceID [-] : Inport  Port=5
  Bus Creator : BusCreator  Inputs='Intensity','Position','Orientation','Color','TextureResourceID'  OutDataTypeStr=Bus: PRESCAN_VISULIGHTACTUATOR_DATA  NonVirtualBus=on
  Bus Creator1 : BusCreator  Inputs=3  OutDataTypeStr=Bus: PRESCAN_RGB_DATA  NonVirtualBus=on
  Bus Creator2 : BusCreator  Inputs=3  OutDataTypeStr=Bus: PRESCAN_RPY_DATA  NonVirtualBus=on
  Bus Creator3 : BusCreator  Inputs=3  OutDataTypeStr=Bus: PRESCAN_XYZ_DATA  NonVirtualBus=on
  Data Type Conversion : DataTypeConversion  OutDataTypeStr=int32  RndMeth=Nearest
  Degrees to Radians : simulink_extras/Transformations/Degrees to Radians
  Demux : Demux  Outputs=3
  Demux1 : Demux  Outputs=3
  Demux2 : Demux  Outputs=3
  Lights : Outport
  wires:
  TextureResourceID [-]/1 -> Data Type Conversion/1  "TextureResourceID"
  MSCD [Cd]/1 -> Bus Creator/1  "Intensity"
  Bus Creator/1 -> Lights/1
  Demux/1 -> Bus Creator1/1  "R"
  Demux/2 -> Bus Creator1/2  "G"
  Demux/3 -> Bus Creator1/3  "B"
  Color [-]/1 -> Demux/1  "Color"
  Bus Creator1/1 -> Bus Creator/4  "Color"
  Demux1/1 -> Bus Creator2/1  "Roll"
  Demux1/2 -> Bus Creator2/2  "Pitch"
  Demux1/3 -> Bus Creator2/3  "Yaw"
  Orientation (RPY) [deg]/1 -> Degrees to Radians/1  "Orientation"
  Bus Creator2/1 -> Bus Creator/3  "Orientation"
  Demux2/1 -> Bus Creator3/1  "X"
  Demux2/2 -> Bus Creator3/2  "Y"
  Demux2/3 -> Bus Creator3/3  "Z"
  Position (xyz) [m]/1 -> Demux2/1  "Position"
  Bus Creator3/1 -> Bus Creator/2  "Position"
  Data Type Conversion/1 -> Bus Creator/5  "TextureResourceID"
  Degrees to Radians/1 -> Demux1/1

== system ACC_speed_change_curve_cs/Audi_A8_1/Brake_light_right_Mux ==
  MSCD [Cd] : Inport
  Position (xyz) [m] : Inport  Port=2
  Orientation (RPY) [deg] : Inport  Port=3
  Color [-] : Inport  Port=4
  TextureResourceID [-] : Inport  Port=5
  Bus Creator : BusCreator  Inputs='Intensity','Position','Orientation','Color','TextureResourceID'  OutDataTypeStr=Bus: PRESCAN_VISULIGHTACTUATOR_DATA  NonVirtualBus=on
  Bus Creator1 : BusCreator  Inputs=3  OutDataTypeStr=Bus: PRESCAN_RGB_DATA  NonVirtualBus=on
  Bus Creator2 : BusCreator  Inputs=3  OutDataTypeStr=Bus: PRESCAN_RPY_DATA  NonVirtualBus=on
  Bus Creator3 : BusCreator  Inputs=3  OutDataTypeStr=Bus: PRESCAN_XYZ_DATA  NonVirtualBus=on
  Data Type Conversion : DataTypeConversion  OutDataTypeStr=int32  RndMeth=Nearest
  Degrees to Radians : simulink_extras/Transformations/Degrees to Radians
  Demux : Demux  Outputs=3
  Demux1 : Demux  Outputs=3
  Demux2 : Demux  Outputs=3
  Lights : Outport
  wires:
  TextureResourceID [-]/1 -> Data Type Conversion/1  "TextureResourceID"
  MSCD [Cd]/1 -> Bus Creator/1  "Intensity"
  Bus Creator/1 -> Lights/1
  Demux/1 -> Bus Creator1/1  "R"
  Demux/2 -> Bus Creator1/2  "G"
  Demux/3 -> Bus Creator1/3  "B"
  Color [-]/1 -> Demux/1  "Color"
  Bus Creator1/1 -> Bus Creator/4  "Color"
  Demux1/1 -> Bus Creator2/1  "Roll"
  Demux1/2 -> Bus Creator2/2  "Pitch"
  Demux1/3 -> Bus Creator2/3  "Yaw"
  Orientation (RPY) [deg]/1 -> Degrees to Radians/1  "Orientation"
  Bus Creator2/1 -> Bus Creator/3  "Orientation"
  Demux2/1 -> Bus Creator3/1  "X"
  Demux2/2 -> Bus Creator3/2  "Y"
  Demux2/3 -> Bus Creator3/3  "Z"
  Position (xyz) [m]/1 -> Demux2/1  "Position"
  Bus Creator3/1 -> Bus Creator/2  "Position"
  Data Type Conversion/1 -> Bus Creator/5  "TextureResourceID"
  Degrees to Radians/1 -> Demux1/1

== system ACC_speed_change_curve_cs/Audi_A8_1/CarSim2PreScan ==
  CarSim_In : Inport
  Ax : Scope
  D2R : Gain  Gain=pi/180
  Demux : Demux  Outputs=[3 3 3 12 1 1 1 1]
  Gain : Gain  Gain=10
  Gain1 : Gain  Gain=9.8
  Mux1 : Mux  Inputs=3
  Transformation_SprungMassdSPACE2PreScan : Subsystem
  Transformation_WheelGlobal2WheelLocal : Subsystem
  km|h_to_m|s : Gain  Gain=1/3.6
  STATE : Outport
  Steer Angle Front [deg] : Outport  Port=2
  zDispl FL[m] : Outport  Port=3
  zDispl FR[m] : Outport  Port=4
  zDispl RL[m] : Outport  Port=5
  zDispl RR[m] : Outport  Port=6
  brake_bar : Outport  Port=7
  Engine_rpm : Outport  Port=8
  Ax_ms-1 : Outport  Port=9
  wires:
  Transformation_SprungMassdSPACE2PreScan/1(Out1) -> Transformation_WheelGlobal2WheelLocal/1(SprungMass_Pos_Global_xyz_[m]), Mux1/1
  Demux/1 -> Transformation_SprungMassdSPACE2PreScan/1(In1)
  Transformation_WheelGlobal2WheelLocal/4(zDispl RR[m]) -> zDispl RR[m]/1
  Transformation_WheelGlobal2WheelLocal/3(zDispl RL[m]) -> zDispl RL[m]/1
  Transformation_WheelGlobal2WheelLocal/2(zDispl FR[m]) -> zDispl FR[m]/1
  Transformation_WheelGlobal2WheelLocal/1(zDispl FL[m]) -> zDispl FL[m]/1
  Demux/5 -> Steer Angle Front [deg]/1
  Mux1/1 -> STATE/1
  CarSim_In/1 -> Demux/1
  km|h_to_m|s/1 -> Mux1/2
  Demux/2 -> km|h_to_m|s/1
  Demux/3 -> D2R/1
  Demux/4 -> Transformation_WheelGlobal2WheelLocal/3(Wheels_Pos_Global_xyz_[m])
  D2R/1 -> Transformation_WheelGlobal2WheelLocal/2(SprungMass_Angle_Global[deg]), Mux1/3
  Demux/6 -> Gain/1
  Demux/7 -> Engine_rpm/1
  Gain/1 -> brake_bar/1
  Demux/8 -> Gain1/1
  Gain1/1 -> Ax/1, Ax_ms-1/1

== system ACC_speed_change_curve_cs/Audi_A8_1/Indicator_front_left_Mux ==
  MSCD [Cd] : Inport
  Position (xyz) [m] : Inport  Port=2
  Orientation (RPY) [deg] : Inport  Port=3
  Color [-] : Inport  Port=4
  TextureResourceID [-] : Inport  Port=5
  Bus Creator : BusCreator  Inputs='Intensity','Position','Orientation','Color','TextureResourceID'  OutDataTypeStr=Bus: PRESCAN_VISULIGHTACTUATOR_DATA  NonVirtualBus=on
  Bus Creator1 : BusCreator  Inputs=3  OutDataTypeStr=Bus: PRESCAN_RGB_DATA  NonVirtualBus=on
  Bus Creator2 : BusCreator  Inputs=3  OutDataTypeStr=Bus: PRESCAN_RPY_DATA  NonVirtualBus=on
  Bus Creator3 : BusCreator  Inputs=3  OutDataTypeStr=Bus: PRESCAN_XYZ_DATA  NonVirtualBus=on
  Data Type Conversion : DataTypeConversion  OutDataTypeStr=int32  RndMeth=Nearest
  Degrees to Radians : simulink_extras/Transformations/Degrees to Radians
  Demux : Demux  Outputs=3
  Demux1 : Demux  Outputs=3
  Demux2 : Demux  Outputs=3
  Lights : Outport
  wires:
  TextureResourceID [-]/1 -> Data Type Conversion/1  "TextureResourceID"
  MSCD [Cd]/1 -> Bus Creator/1  "Intensity"
  Bus Creator/1 -> Lights/1
  Demux/1 -> Bus Creator1/1  "R"
  Demux/2 -> Bus Creator1/2  "G"
  Demux/3 -> Bus Creator1/3  "B"
  Color [-]/1 -> Demux/1  "Color"
  Bus Creator1/1 -> Bus Creator/4  "Color"
  Demux1/1 -> Bus Creator2/1  "Roll"
  Demux1/2 -> Bus Creator2/2  "Pitch"
  Demux1/3 -> Bus Creator2/3  "Yaw"
  Orientation (RPY) [deg]/1 -> Degrees to Radians/1  "Orientation"
  Bus Creator2/1 -> Bus Creator/3  "Orientation"
  Demux2/1 -> Bus Creator3/1  "X"
  Demux2/2 -> Bus Creator3/2  "Y"
  Demux2/3 -> Bus Creator3/3  "Z"
  Position (xyz) [m]/1 -> Demux2/1  "Position"
  Bus Creator3/1 -> Bus Creator/2  "Position"
  Data Type Conversion/1 -> Bus Creator/5  "TextureResourceID"
  Degrees to Radians/1 -> Demux1/1

== system ACC_speed_change_curve_cs/Audi_A8_1/Indicator_front_right_Mux ==
  MSCD [Cd] : Inport
  Position (xyz) [m] : Inport  Port=2
  Orientation (RPY) [deg] : Inport  Port=3
  Color [-] : Inport  Port=4
  TextureResourceID [-] : Inport  Port=5
  Bus Creator : BusCreator  Inputs='Intensity','Position','Orientation','Color','TextureResourceID'  OutDataTypeStr=Bus: PRESCAN_VISULIGHTACTUATOR_DATA  NonVirtualBus=on
  Bus Creator1 : BusCreator  Inputs=3  OutDataTypeStr=Bus: PRESCAN_RGB_DATA  NonVirtualBus=on
  Bus Creator2 : BusCreator  Inputs=3  OutDataTypeStr=Bus: PRESCAN_RPY_DATA  NonVirtualBus=on
  Bus Creator3 : BusCreator  Inputs=3  OutDataTypeStr=Bus: PRESCAN_XYZ_DATA  NonVirtualBus=on
  Data Type Conversion : DataTypeConversion  OutDataTypeStr=int32  RndMeth=Nearest
  Degrees to Radians : simulink_extras/Transformations/Degrees to Radians
  Demux : Demux  Outputs=3
  Demux1 : Demux  Outputs=3
  Demux2 : Demux  Outputs=3
  Lights : Outport
  wires:
  TextureResourceID [-]/1 -> Data Type Conversion/1  "TextureResourceID"
  MSCD [Cd]/1 -> Bus Creator/1  "Intensity"
  Bus Creator/1 -> Lights/1
  Demux/1 -> Bus Creator1/1  "R"
  Demux/2 -> Bus Creator1/2  "G"
  Demux/3 -> Bus Creator1/3  "B"
  Color [-]/1 -> Demux/1  "Color"
  Bus Creator1/1 -> Bus Creator/4  "Color"
  Demux1/1 -> Bus Creator2/1  "Roll"
  Demux1/2 -> Bus Creator2/2  "Pitch"
  Demux1/3 -> Bus Creator2/3  "Yaw"
  Orientation (RPY) [deg]/1 -> Degrees to Radians/1  "Orientation"
  Bus Creator2/1 -> Bus Creator/3  "Orientation"
  Demux2/1 -> Bus Creator3/1  "X"
  Demux2/2 -> Bus Creator3/2  "Y"
  Demux2/3 -> Bus Creator3/3  "Z"
  Position (xyz) [m]/1 -> Demux2/1  "Position"
  Bus Creator3/1 -> Bus Creator/2  "Position"
  Data Type Conversion/1 -> Bus Creator/5  "TextureResourceID"
  Degrees to Radians/1 -> Demux1/1

== system ACC_speed_change_curve_cs/Audi_A8_1/Indicator_rear_left_Mux ==
  MSCD [Cd] : Inport
  Position (xyz) [m] : Inport  Port=2
  Orientation (RPY) [deg] : Inport  Port=3
  Color [-] : Inport  Port=4
  TextureResourceID [-] : Inport  Port=5
  Bus Creator : BusCreator  Inputs='Intensity','Position','Orientation','Color','TextureResourceID'  OutDataTypeStr=Bus: PRESCAN_VISULIGHTACTUATOR_DATA  NonVirtualBus=on
  Bus Creator1 : BusCreator  Inputs=3  OutDataTypeStr=Bus: PRESCAN_RGB_DATA  NonVirtualBus=on
  Bus Creator2 : BusCreator  Inputs=3  OutDataTypeStr=Bus: PRESCAN_RPY_DATA  NonVirtualBus=on
  Bus Creator3 : BusCreator  Inputs=3  OutDataTypeStr=Bus: PRESCAN_XYZ_DATA  NonVirtualBus=on
  Data Type Conversion : DataTypeConversion  OutDataTypeStr=int32  RndMeth=Nearest
  Degrees to Radians : simulink_extras/Transformations/Degrees to Radians
  Demux : Demux  Outputs=3
  Demux1 : Demux  Outputs=3
  Demux2 : Demux  Outputs=3
  Lights : Outport
  wires:
  TextureResourceID [-]/1 -> Data Type Conversion/1  "TextureResourceID"
  MSCD [Cd]/1 -> Bus Creator/1  "Intensity"
  Bus Creator/1 -> Lights/1
  Demux/1 -> Bus Creator1/1  "R"
  Demux/2 -> Bus Creator1/2  "G"
  Demux/3 -> Bus Creator1/3  "B"
  Color [-]/1 -> Demux/1  "Color"
  Bus Creator1/1 -> Bus Creator/4  "Color"
  Demux1/1 -> Bus Creator2/1  "Roll"
  Demux1/2 -> Bus Creator2/2  "Pitch"
  Demux1/3 -> Bus Creator2/3  "Yaw"
  Orientation (RPY) [deg]/1 -> Degrees to Radians/1  "Orientation"
  Bus Creator2/1 -> Bus Creator/3  "Orientation"
  Demux2/1 -> Bus Creator3/1  "X"
  Demux2/2 -> Bus Creator3/2  "Y"
  Demux2/3 -> Bus Creator3/3  "Z"
  Position (xyz) [m]/1 -> Demux2/1  "Position"
  Bus Creator3/1 -> Bus Creator/2  "Position"
  Data Type Conversion/1 -> Bus Creator/5  "TextureResourceID"
  Degrees to Radians/1 -> Demux1/1

== system ACC_speed_change_curve_cs/Audi_A8_1/Indicator_rear_right_Mux ==
  MSCD [Cd] : Inport
  Position (xyz) [m] : Inport  Port=2
  Orientation (RPY) [deg] : Inport  Port=3
  Color [-] : Inport  Port=4
  TextureResourceID [-] : Inport  Port=5
  Bus Creator : BusCreator  Inputs='Intensity','Position','Orientation','Color','TextureResourceID'  OutDataTypeStr=Bus: PRESCAN_VISULIGHTACTUATOR_DATA  NonVirtualBus=on
  Bus Creator1 : BusCreator  Inputs=3  OutDataTypeStr=Bus: PRESCAN_RGB_DATA  NonVirtualBus=on
  Bus Creator2 : BusCreator  Inputs=3  OutDataTypeStr=Bus: PRESCAN_RPY_DATA  NonVirtualBus=on
  Bus Creator3 : BusCreator  Inputs=3  OutDataTypeStr=Bus: PRESCAN_XYZ_DATA  NonVirtualBus=on
  Data Type Conversion : DataTypeConversion  OutDataTypeStr=int32  RndMeth=Nearest
  Degrees to Radians : simulink_extras/Transformations/Degrees to Radians
  Demux : Demux  Outputs=3
  Demux1 : Demux  Outputs=3
  Demux2 : Demux  Outputs=3
  Lights : Outport
  wires:
  TextureResourceID [-]/1 -> Data Type Conversion/1  "TextureResourceID"
  MSCD [Cd]/1 -> Bus Creator/1  "Intensity"
  Bus Creator/1 -> Lights/1
  Demux/1 -> Bus Creator1/1  "R"
  Demux/2 -> Bus Creator1/2  "G"
  Demux/3 -> Bus Creator1/3  "B"
  Color [-]/1 -> Demux/1  "Color"
  Bus Creator1/1 -> Bus Creator/4  "Color"
  Demux1/1 -> Bus Creator2/1  "Roll"
  Demux1/2 -> Bus Creator2/2  "Pitch"
  Demux1/3 -> Bus Creator2/3  "Yaw"
  Orientation (RPY) [deg]/1 -> Degrees to Radians/1  "Orientation"
  Bus Creator2/1 -> Bus Creator/3  "Orientation"
  Demux2/1 -> Bus Creator3/1  "X"
  Demux2/2 -> Bus Creator3/2  "Y"
  Demux2/3 -> Bus Creator3/3  "Z"
  Position (xyz) [m]/1 -> Demux2/1  "Position"
  Bus Creator3/1 -> Bus Creator/2  "Position"
  Data Type Conversion/1 -> Bus Creator/5  "TextureResourceID"
  Degrees to Radians/1 -> Demux1/1

== system ACC_speed_change_curve_cs/Audi_A8_1/JointGroup_WheelDisplacement_V2R ==
  Velocity [m/s] : Inport  SampleTime=TimeStep
  Discrete-Time Integrator : DiscreteIntegrator  SampleTime=TimeStep  ICPrevOutput=DiscIntNeverNeededParam  ICPrevScaledInput=DiscIntNeverNeededParam
  omega=V/Rwheel : Gain  Gain=1/TireRadius
  Rotation [rad] : Outport
  wires:
  Discrete-Time Integrator/1 -> Rotation [rad]/1  "roty"
  omega=V/Rwheel/1 -> Discrete-Time Integrator/1  "rotational speed [rad/s]"
  Velocity [m/s]/1 -> omega=V/Rwheel/1

== system ACC_speed_change_curve_cs/Audi_A8_1/PathFollower_1 ==
  TrajOffset_x,y,Y [m,m,deg] : Inport
  ActorOffset_Left(+) / Right(-) [m] : Inport  Port=2
  position x,y,Y [m,m,deg] : Inport  Port=3
  Initial Velocity [m/s] : Inport  Port=4
  Desired Velocity [m/s] : Inport  Port=5
  velocity [m/s] : Inport  Port=6
  CTRL REFERENCES : Subsystem
  Calculate shifted p0 wrt COG : Subsystem
  DELTA CTRL : Subsystem
  Demux : Demux  Outputs=3
  Gain : Gain  Gain=1*pi/180
  Goto Tag Visibility : GotoTagVisibility  GotoTag=PreviewDistance
  Goto Tag Visibility1 : GotoTagVisibility  GotoTag=v_actual
  Memory1 : Memory
  Memory2 : Memory
  Memory3 : Memory
  Mux : Mux  Inputs=3
  Preview distance velocity dependent : Lookup  InputValues=[0 20 30 40 50 60 70 80 90 100 120]  Table=[1 1 2 3 4 5 6 7 10 13.33 20]
  THROTTLE CTRL : Subsystem
  sign1 : Gain  Gain=3.6
  delta_steerwheel [deg] : Outport
  throttle [%] : Outport  Port=2
  brake pressure [bar] : Outport  Port=3
  v0 [m/s] : Outport  Port=4
  Auto_GearShift : Outport  Port=5
  Actor/Traj_distance [m] : Outport  Port=6
  Actor/Traj_angle [deg] : Outport  Port=7
  tag scope: PreviewDistance=scoped, v_actual=scoped
  wires:
  Memory3/1 -> CTRL REFERENCES/4(ActorOffset_Left(+) / Right(-)_[m])
  THROTTLE CTRL/4(Auto_GearShift) -> Auto_GearShift/1
  THROTTLE CTRL/2(brake pressure [bar]) -> brake pressure [bar]/1
  Memory2/1 -> THROTTLE CTRL/1(v_actual [m/s]), [v_actual]
  Memory1/1 -> DELTA CTRL/1(p0), CTRL REFERENCES/1(Pos x,y,Y [m,m,rad])
  sign1/1 -> Preview distance velocity dependent/1
  Initial Velocity [m/s]/1 -> THROTTLE CTRL/3(Initial Velocity [m/s])
  velocity [m/s]/1 -> Memory2/1
  CTRL REFERENCES/1(pvp  [m,m]) -> DELTA CTRL/2(pvp)
  CTRL REFERENCES/2(pref_pvp [m,m]) -> DELTA CTRL/3(pref_pvp)
  Gain/1 -> Mux/3
  DELTA CTRL/1(delta_steerwheel [deg]) -> delta_steerwheel [deg]/1
  Mux/1 -> CTRL REFERENCES/3(TrajOffset [m,m,rad])
  CTRL REFERENCES/3(pref_0 [m,m]) -> DELTA CTRL/4(pref0)
  THROTTLE CTRL/3(v0 [m/s]) -> v0 [m/s]/1
  THROTTLE CTRL/1(throttle [%]) -> throttle [%]/1
  [v_actual] -> sign1/1
  Preview distance velocity dependent/1 -> [PreviewDistance], CTRL REFERENCES/2(Position Preview Distance [m])
  Desired Velocity [m/s]/1 -> THROTTLE CTRL/2(Desired Velocity [m/s])
  ActorOffset_Left(+) / Right(-) [m]/1 -> Memory3/1
  Demux/1 -> Mux/1
  Demux/2 -> Mux/2
  Demux/3 -> Gain/1
  TrajOffset_x,y,Y [m,m,deg]/1 -> Demux/1
  Calculate shifted p0 wrt COG/1(position x,y,Y [m,m,rad]) -> Memory1/1
  position x,y,Y [m,m,deg]/1 -> Calculate shifted p0 wrt COG/1(position x,y,Y [m,m,deg])
  CTRL REFERENCES/4(Actor/Traj_distance [m]) -> Actor/Traj_distance [m]/1
  CTRL REFERENCES/5(Actor/Traj_angle [deg]) -> Actor/Traj_angle [deg]/1

== system ACC_speed_change_curve_cs/Audi_A8_1/SELF_Demux ==
  SELF : Inport  OutDataTypeStr=Bus: PRESCAN_SELFSENSORDATA
  Bus Selector : BusSelector  OutputSignals=PositionX,PositionY,PositionZ,OrientationRoll,OrientationPitch,OrientationYaw,Velocity,Yaw_rate,Lat,Long,Alt
  Demux2 : Demux  Outputs=3
  Gain : Gain  Gain=180/pi
  Gain1 : Gain  Gain=180/pi
  Vector Concatenate1 : Concatenate  NumInputs=3
  compas converter : Subsystem
  x [m] : Outport
  y [m] : Outport  Port=2
  z [m] : Outport  Port=3
  rotx [deg] : Outport  Port=4
  roty [deg] : Outport  Port=5
  rotz [deg] : Outport  Port=6
  GPS lat [deg] : Outport  Port=7
  GPS long [deg] : Outport  Port=8
  GPS alt [m] : Outport  Port=9
  velocity [m/s] : Outport  Port=10
  heading [deg] : Outport  Port=11
  yaw rate [deg/s] : Outport  Port=12
  wires:
  Bus Selector/11 -> GPS alt [m]/1  "<Alt>"
  Bus Selector/10 -> GPS long [deg]/1  "<Long>"
  Bus Selector/9 -> GPS lat [deg]/1  "<Lat>"
  Bus Selector/8 -> Gain1/1  "<Yaw_rate>"
  Bus Selector/7 -> velocity [m/s]/1  "<Velocity>"
  Bus Selector/6 -> compas converter/1(rotz [rad]), Vector Concatenate1/3  "<OrientationYaw>"
  Bus Selector/5 -> Vector Concatenate1/2  "<OrientationPitch>"
  Bus Selector/4 -> Vector Concatenate1/1  "<OrientationRoll>"
  Vector Concatenate1/1 -> Gain/1
  Bus Selector/3 -> z [m]/1  "<PositionZ>"
  Bus Selector/2 -> y [m]/1  "<PositionY>"
  Bus Selector/1 -> x [m]/1  "<PositionX>"
  SELF/1 -> Bus Selector/1
  Gain/1 -> Demux2/1
  Demux2/1 -> rotx [deg]/1
  Demux2/2 -> roty [deg]/1
  Demux2/3 -> rotz [deg]/1
  compas converter/1(heading [deg]) -> heading [deg]/1
  Gain1/1 -> yaw rate [deg/s]/1

== system ACC_speed_change_curve_cs/Audi_A8_1/STATE_Audi_A8_1 ==
  State : Inport  SampleTime=TimeStep
  Bus Creator : BusCreator  Inputs=15  OutDataTypeStr=Bus: PRESCAN_STATEACTUATORDATA  NonVirtualBus=on
  Demux : Demux  Outputs=15
  iniBODYAngles wrtVEH [rad] : Constant  Value=[Roll0 Pitch0 0]  SampleTime=TimeStep
  iniVEHAngles wrtGLOB [rad] : Constant  Value=[0 0 Yaw0]  SampleTime=TimeStep
  iniVEHposition wrtGLOB [m] : Constant  Value=[x0 y0 z0]  SampleTime=TimeStep
  state2FullState : PreScanSimulinkLibrary/state2FullState  SystemSampleTime=-1
  StateBus : Outport  OutDataTypeStr=Bus: PRESCAN_STATEACTUATORDATA
  wires:
  Bus Creator/1 -> StateBus/1
  State/1 -> state2FullState/1
  state2FullState/1 -> Demux/1
  iniVEHposition wrtGLOB [m]/1 -> state2FullState/2
  iniBODYAngles wrtVEH [rad]/1 -> state2FullState/3
  iniVEHAngles wrtGLOB [rad]/1 -> state2FullState/4
  Demux/1 -> Bus Creator/1  "PositionX"
  Demux/2 -> Bus Creator/2  "PositionY"
  Demux/3 -> Bus Creator/3  "PositionZ"
  Demux/4 -> Bus Creator/4  "VelocityX"
  Demux/5 -> Bus Creator/5  "VelocityY"
  Demux/6 -> Bus Creator/6  "VelocityZ"
  Demux/7 -> Bus Creator/7  "AccelerationX"
  Demux/8 -> Bus Creator/8  "AccelerationY"
  Demux/9 -> Bus Creator/9  "AccelerationZ"
  Demux/10 -> Bus Creator/10  "OrientationRoll"
  Demux/11 -> Bus Creator/11  "OrientationPitch"
  Demux/12 -> Bus Creator/12  "OrientationYaw"
  Demux/13 -> Bus Creator/13  "AngularVelocityRoll"
  Demux/14 -> Bus Creator/14  "AngularVelocityPitch"
  Demux/15 -> Bus Creator/15  "AngularVelocityYaw"
